simulink model "WalecOstroslup"  (R2022b)
settings: Solver=VariableStepAuto  StartTime=0.0  StopTime=200  RelTol=1e-3
values from neighbouring files (symbols this model uses):
  a2 = 3.59153    [Lab_3.m]    (also in PA_Lab3.m)
  b2 = 7.79612    [Lab_3.m]    (also in PA_Lab3.m)
  c1 = 4.3589    [Lab_3.m]    (also in PA_Lab3.m)
  c2 = 3.08221    [Lab_3.m]    (also in PA_Lab3.m)
  h1i = 0    [Lab_3.m]    (also in PA_Lab3.m = 0.949998151594)
  H2 = 19    [Lab_3.m]    (also in PA_Lab3.m)
  h20 = (qwe/c2)^2    (= 9.49998151594)    [Lab_3.m]    (also in PA_Lab3.m)
  h2i = 0.1*h20    (= 0.949998151594)    [Lab_3.m]    (also in PA_Lab3.m)
  kr = 5.2928    [Lab_3.m]    (also in PA_Lab3.m = kra)
  qwe = 0.5*H2    (= 9.5)    [Lab_3.m]    (also in PA_Lab3.m)
  R1 = 1.12838    [Lab_3.m]    (also in PA_Lab3.m)
  T3 = 0.3*min(T1, T2)    [Lab_3.m]    (also in PA_Lab3.m = 0.2*min(T1, T2))
undefined symbols (not defined in the file or in its folder): L, M
settings Model: Creator=Gabriel  LastModifiedBy=barte
settings SolverCC: InitialStep=10^-6
settings DataIOCC: ReturnWorkspaceOutputs=off

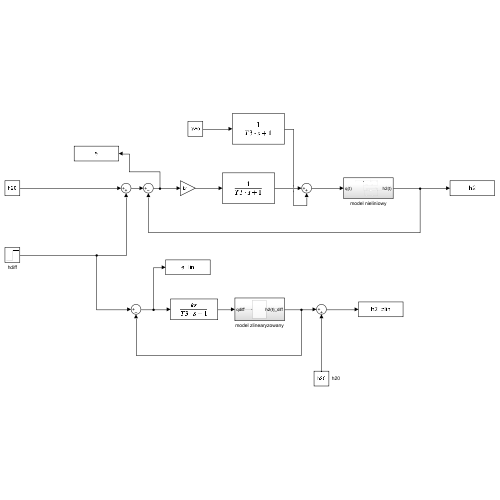
[thumbnail: Simulink's stored preview of the top-level diagram]
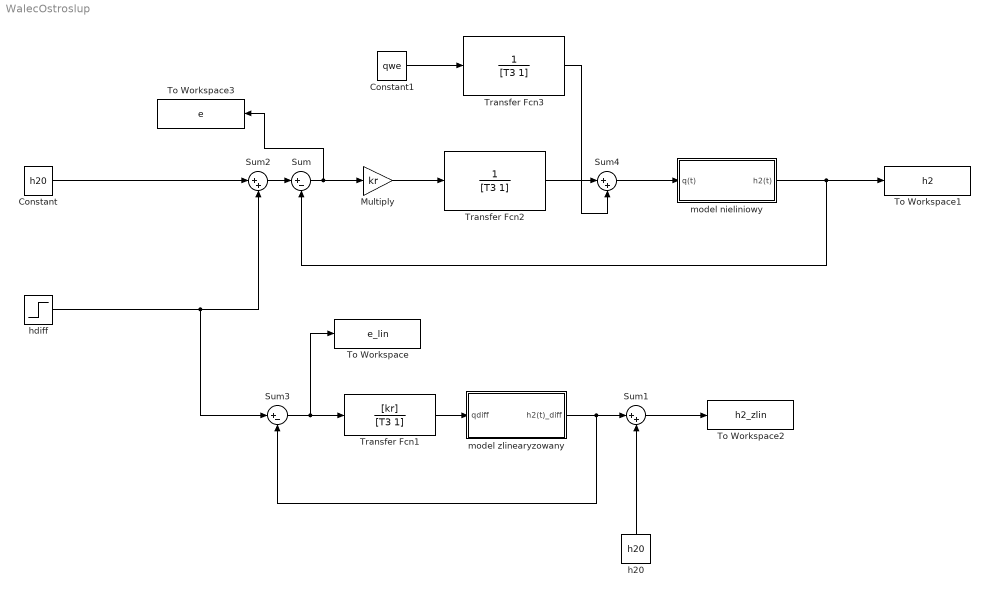
== system WalecOstroslup ==
  Constant : Constant  Value=h20
  Constant1 : Constant  Value=qwe
  Multiply : Gain  Gain=kr
  Sum : Sum  Inputs=|+-
  Sum1 : Sum  Inputs=|++
  Sum2 : Sum  Inputs=|++
  Sum3 : Sum  Inputs=|+-
  Sum4 : Sum  Inputs=|++
  To Workspace : ToWorkspace  VariableName=e_lin  SaveFormat=Timeseries  SampleTime=10^-3
  To Workspace1 : ToWorkspace  VariableName=h2  SaveFormat=Timeseries  SampleTime=10^-3
  To Workspace2 : ToWorkspace  VariableName=h2_zlin  SaveFormat=Timeseries  SampleTime=10^-3
  To Workspace3 : ToWorkspace  VariableName=e  SaveFormat=Timeseries  SampleTime=-1
  Transfer Fcn1 : TransferFcn  Numerator=[kr]  Denominator=[T3 1]
  Transfer Fcn2 : TransferFcn  Denominator=[T3 1]
  Transfer Fcn3 : TransferFcn  Denominator=[T3 1]
  h20 : Constant  Value=h20
  hdiff : Step  Time=120  After=0.05*h20  SampleTime=0
  model nieliniowy : Subsystem
  model zlinearyzowany : Subsystem
  wires:
  model zlinearyzowany/1(h2(t)_diff) -> Sum3/2, Sum1/1
  h20/1 -> Sum1/2
  Sum1/1 -> To Workspace2/1
  Transfer Fcn1/1 -> model zlinearyzowany/1(qdiff)
  Sum3/1 -> To Workspace/1, Transfer Fcn1/1
  hdiff/1 -> Sum2/2, Sum3/1
  Constant/1 -> Sum2/1
  model nieliniowy/1(h2(t)) -> Sum/2, To Workspace1/1
  Sum2/1 -> Sum/1
  Sum/1 -> Multiply/1, To Workspace3/1
  Multiply/1 -> Transfer Fcn2/1
  Transfer Fcn2/1 -> Sum4/1
  Sum4/1 -> model nieliniowy/1(q(t))
  Constant1/1 -> Transfer Fcn3/1
  Transfer Fcn3/1 -> Sum4/2

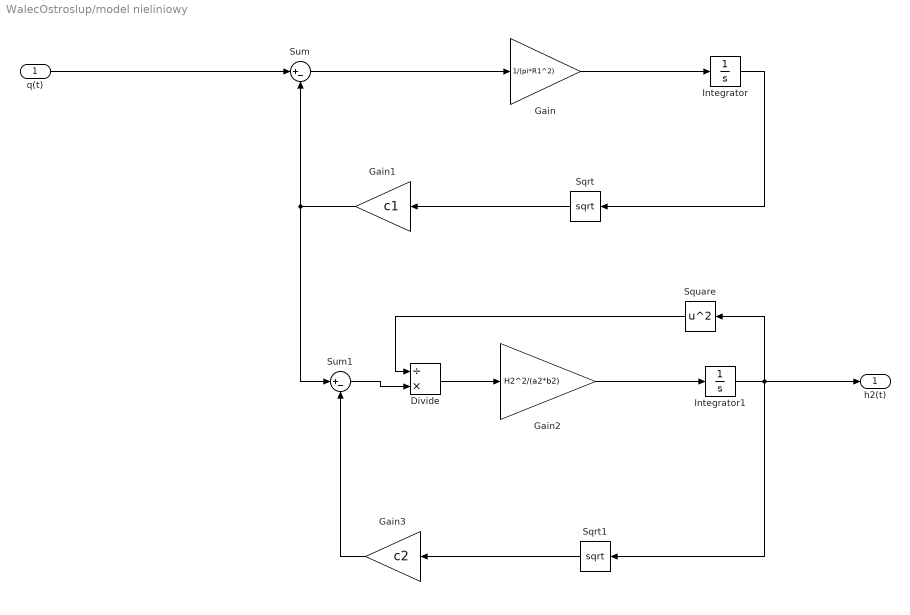
== system WalecOstroslup/model nieliniowy ==
  q(t) : Inport
  Divide : Product  Inputs=/*
  Gain : Gain  Gain=1/(pi*R1^2)
  Gain1 : Gain  Gain=c1
  Gain2 : Gain  Gain=H2^2/(a2*b2)
  Gain3 : Gain  Gain=c2
  Integrator : Integrator  InitialCondition=h1i
  Integrator1 : Integrator  InitialCondition=h2i
  Sqrt : Sqrt
  Sqrt1 : Sqrt
  Square : Math  Operator=square
  Sum : Sum  Inputs=|+-
  Sum1 : Sum  Inputs=|+-
  h2(t) : Outport
  wires:
  Gain1/1 -> Sum/2, Sum1/1
  Sum/1 -> Gain/1
  Sqrt/1 -> Gain1/1
  Integrator1/1 -> h2(t)/1, Square/1, Sqrt1/1
  Square/1 -> Divide/1
  Gain2/1 -> Integrator1/1
  Gain/1 -> Integrator/1
  Divide/1 -> Gain2/1
  Gain3/1 -> Sum1/2
  Sqrt1/1 -> Gain3/1
  Sum1/1 -> Divide/2
  q(t)/1 -> Sum/1
  Integrator/1 -> Sqrt/1

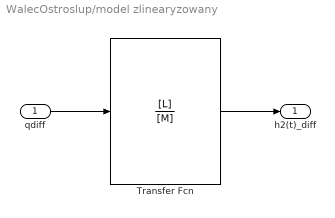
== system WalecOstroslup/model zlinearyzowany ==
  qdiff : Inport
  Transfer Fcn : TransferFcn  Numerator=[L]  Denominator=[M]
  h2(t)_diff : Outport
  wires:
  Transfer Fcn/1 -> h2(t)_diff/1
  qdiff/1 -> Transfer Fcn/1
